simulink model "trans_line_1"  (Simulink 7.4)
settings: Solver=ode45  StartTime=0.0  StopTime=1e-7  MaxStep=1e-9;  RelTol=1e-3
PreLoadFcn:
  | cpf=28e-12;    % cap per ft of typical 50 ohm line
  | c    = 3e8;         % speed of light
  | Zo = 50;
  | lpf = cpf* (Zo^2);
  | 
  | kmpft = (12/39.42)*.001; % kilometers per ft
libraries: powerlib x12, simulink x3
settings Model: Creator=dbenson  LastModifiedBy=Dick
settings OptimizationCC: InitFltsAndDblsToZero=on
settings DebuggingCC: SaveWithParameterizedLinksMsg=none  SignalResolutionControl=TryResolveAllWithWarning  MultiTaskDSMMsg=warning  MultiTaskCondExecSysMsg=none
settings RTWCC: IncludeERTFirstTime=on
settings GRTTargetCC: TargetFcnLib=ansi_tfl_tmw.mat

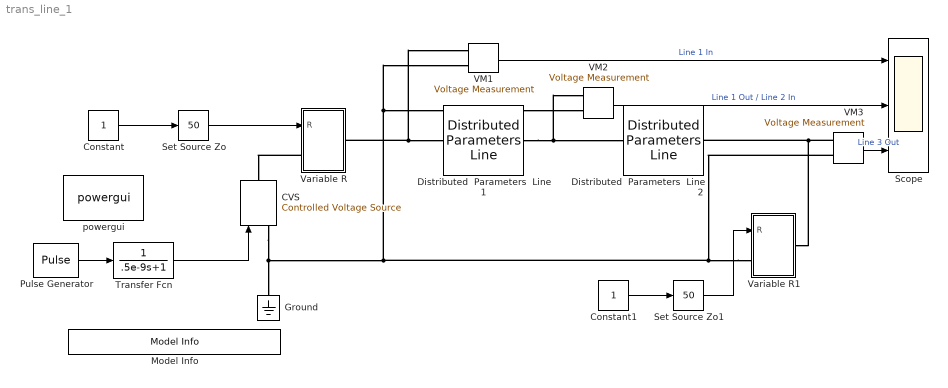
== system trans_line_1 ==
  CVS : powerlib/Electrical Sources/Controlled Voltage Source  DialogController=POWERSYS.PowerSysDialog  SystemSampleTime=-1  Initialize=off  Source_Type=DC  Amplitude=0  Phase=0  Frequency=0  Measurements=None
  Constant : Constant  OutDataType=sfix(16)  OutScaling=2^0
  Constant1 : Constant  OutDataType=sfix(16)  OutScaling=2^0
  Distributed  Parameters  Line 1 : powerlib/Elements/Distributed Parameters Line  DialogController=POWERSYS.PowerSysDialog  SystemSampleTime=-1  Phases=1  Frequency=1e6  Resistance=[1]  Inductance=lpf/kmpft  Capacitance=cpf/kmpft  Length=.001  x1=[0 0;9.198e-010 0;1.8396e-009 0;2.7594e-009 0;3.6792e-009 0;4.599e-009 0]  x2=[0 0;9.198e-010 0;1.8396e-009 0;2.7594e-009 0;3.6792e-009 0;4.599e-009 0]  x3=[0 0;9.198e-010 0;1.8396e-009 0;2.7594e-009 0;3.6792e-009 0;4.599e-009 0]  x4=[0 0;9.198e-010 0;1.8396e-009 0;2.7594e-009 0;3.6792e-009 0;4.599e-009 0]  x5=4.599e-009  Measurements=None
  Distributed  Parameters  Line 2 : powerlib/Elements/Distributed Parameters Line  DialogController=POWERSYS.PowerSysDialog  SystemSampleTime=-1  Phases=1  Frequency=1e6  Resistance=[1]  Inductance=lpf/kmpft  Capacitance=cpf/kmpft  Length=.001  x1=[0 0;9.198e-010 0;1.8396e-009 0;2.7594e-009 0;3.6792e-009 0;4.599e-009 0]  x2=[0 0;9.198e-010 0;1.8396e-009 0;2.7594e-009 0;3.6792e-009 0;4.599e-009 0]  x3=[0 0;9.198e-010 0;1.8396e-009 0;2.7594e-009 0;3.6792e-009 0;4.599e-009 0]  x4=[0 0;9.198e-010 0;1.8396e-009 0;2.7594e-009 0;3.6792e-009 0;4.599e-009 0]  x5=4.599e-009  Measurements=None
  Ground : powerlib/Elements/Ground  DialogController=POWERSYS.PowerSysDialog  PhysicalDomain=powersysdomain  SubClassName=unknown  LeftPortType=p1  RightPortType=p1  LConnTagsString=a
  Model Info : simulink/Model-Wide Utilities/Model Info  SystemSampleTime=-1  InitialBlockCM=None  BlockCM=None  Frame=on  DisplayStringWithTags=Copywrite 2005-2010 The MathWorks, Inc.  HorizontalTextAlignment=Center  LeftAlignmentValue=0.5  SourceBlockDiagram=trans_line_1  TagMaxNumber=20
  Pulse Generator : DiscretePulseGenerator  PulseType=Time based  Amplitude=1  Period=1e-7  PulseWidth=50  PhaseDelay=0  SampleTime=1
  Scope : Scope  NumInputPorts=3
      settings: YMin=-0.5~-0.5~-0.5  YMax=1.5~1.5~1.5
  Set Source Zo : simulink/Math Operations/Slider Gain  SystemSampleTime=-1  low=0  gain=50  high=100
  Set Source Zo1 : simulink/Math Operations/Slider Gain  SystemSampleTime=-1  low=0  gain=50  high=100
  Transfer Fcn : TransferFcn  Denominator=[.5e-9 1]
  VM1 : powerlib/Measurements/Voltage Measurement  DialogController=POWERSYS.PowerSysDialog  SystemSampleTime=-1  PhasorSimulation=off  OutputType=Complex  PSBequivalent=0
  VM2 : powerlib/Measurements/Voltage Measurement  DialogController=POWERSYS.PowerSysDialog  SystemSampleTime=-1  PhasorSimulation=off  OutputType=Complex  PSBequivalent=0
  VM3 : powerlib/Measurements/Voltage Measurement  DialogController=POWERSYS.PowerSysDialog  SystemSampleTime=-1  PhasorSimulation=off  OutputType=Complex  PSBequivalent=0
  Variable R : Subsystem
  Variable R1 : Subsystem
  powergui : powerlib/powergui  SystemSampleTime=-1  SimulationMode=Continuous  SampleTime=50e-6  frequency=60  SPID=off  DisableSnubberDevices=off  DisableRonSwitches=off  DisableVfSwitches=off  SwTol=0  Interpol=off  frequencyindice=0  echomessages=off  HookPort=off  DisplayEquations=off  FunctionMessages=off  EnableUseOfTLC=off  x0status=blocks  RestoreLinks=warning  Frange=[0:2:500]  Ylog=off  Xlog=on  ShowGrid=off  save=off  variable=ZData  ZoomFFT=on  StartTime=0.0  cycles=1  DisplayStyle=1  fundamental=60  FreqAxis=off  MaxFrequency=1000  frequencyindicesteady=1  RmsSteady=1  display=off  Ts=0  methode=off
  wires:
  VM2/1 -> Scope/2  "Line 1 Out / Line 2 In"
  Pulse Generator/1 -> Transfer Fcn/1
  Transfer Fcn/1 -> CVS/1
  VM1/1 -> Scope/1  "Line 1 In"
  VM3/1 -> Scope/3  "Line 3 Out"
  Set Source Zo/1 -> Variable R/1(R)
  Constant/1 -> Set Source Zo/1
  Set Source Zo1/1 -> Variable R1/1(R)
  Constant1/1 -> Set Source Zo1/1
  connections:
  Variable R/RConn1 -- Distributed  Parameters  Line 1/LConn1 -- VM1/LConn1
  Variable R/LConn1 -- CVS/RConn1
  Distributed  Parameters  Line 1/RConn1 -- VM2/LConn1 -- Distributed  Parameters  Line 2/LConn1
  Variable R1/LConn1 -- VM3/LConn2 -- VM1/LConn2 -- VM2/LConn2 -- CVS/LConn1 -- Ground/LConn1
  VM3/LConn1 -- Distributed  Parameters  Line 2/RConn1 -- Variable R1/RConn1

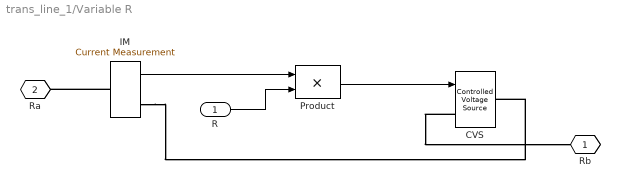
== system trans_line_1/Variable R ==
  R : Inport  OutDataType=sfix(16)  OutScaling=2^0
  CVS : powerlib/Electrical Sources/Controlled Voltage Source  Description=source block  DialogController=POWERSYS.PowerSysDialog  SystemSampleTime=-1  Initialize=off  Source_Type=AC  Amplitude=0  Phase=0  Frequency=0  Measurements=None
      settings: AttributesFormatString=\n
  IM : powerlib/Measurements/Current Measurement  Tag=PoWeRsYsTeMmEaSuReMeNt  DialogController=POWERSYS.PowerSysDialog  SystemSampleTime=-1  PhasorSimulation=off  OutputType=Magnitude  PSBequivalent=0
  Product : Product  Inputs=**  OutDataType=sfix(16)  OutScaling=2^0  SaturateOnIntegerOverflow=on  OutDataTypeStr=Inherit: Same as first input
  Rb : PMIOPort  Tag=PMCPort  Port=1  Side=Right
  Ra : PMIOPort  Tag=PMCPort  Port=2  Side=Left
  wires:
  Product/1 -> CVS/1
  IM/1 -> Product/1
  R/1 -> Product/2
  connections:
  CVS/LConn1 -- Rb/RConn1
  IM/RConn1 -- CVS/RConn1
  IM/LConn1 -- Ra/RConn1

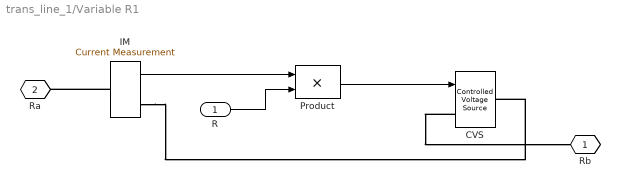
== system trans_line_1/Variable R1 ==
  R : Inport  OutDataType=sfix(16)  OutScaling=2^0
  CVS : powerlib/Electrical Sources/Controlled Voltage Source  Description=source block  DialogController=POWERSYS.PowerSysDialog  SystemSampleTime=-1  Initialize=off  Source_Type=AC  Amplitude=0  Phase=0  Frequency=0  Measurements=None
      settings: AttributesFormatString=\n
  IM : powerlib/Measurements/Current Measurement  Tag=PoWeRsYsTeMmEaSuReMeNt  DialogController=POWERSYS.PowerSysDialog  SystemSampleTime=-1  PhasorSimulation=off  OutputType=Magnitude  PSBequivalent=0
  Product : Product  Inputs=**  OutDataType=sfix(16)  OutScaling=2^0  SaturateOnIntegerOverflow=on  OutDataTypeStr=Inherit: Same as first input
  Rb : PMIOPort  Tag=PMCPort  Port=1  Side=Right
  Ra : PMIOPort  Tag=PMCPort  Port=2  Side=Left
  wires:
  R/1 -> Product/2
  IM/1 -> Product/1
  Product/1 -> CVS/1
  connections:
  IM/LConn1 -- Ra/RConn1
  IM/RConn1 -- CVS/RConn1
  CVS/LConn1 -- Rb/RConn1
